simulink model "project_sim"  (R2022b)
settings: Solver=VariableStepAuto  StartTime=0.0  StopTime=Tf  RelTol=1e-3
values from neighbouring files (symbols this model uses):
  FSW_freq = 1/10    (= 0.1)    [project.m]
  h0 = 4881    [project.m]
  J = J + J'    [TestRK4.m]    (also in project.m = 1E-4*[24181836 3783405 3898808)
  kd_nonlin = 10    [project.m]
  kp_nonlin = 0.1    [project.m]
  mu = 398600    [project.m]
  Phat0 = blkdiag(1E-3*eye(3),1E-4*eye(3))    [project.m]
  Q_filter = blkdiag(1E-8*eye(3),0.1*w_noise_scale*eye(3))    [project.m]
  q_inertial2body_0_est = QuatProduct(dq0_disp,q_inertial2body_0)    [project.m]
  q_inertial2body_0_true = QuatProduct(dq0,q_inertial2body_0_est)    [project.m]
  q_inertial2LVLH_0 = DCM2Quat(T_inertial2LVLH_0)    [project.m]
  q_LVLH2body_0_est = QuatProduct(q_inertial2body_0_est,QuatInv(q_inertial2LVLH_0))    [project.m]
  q_LVLH2body_f = QuatProduct(q_change,q_LVLH2body_0)    [project.m]
  rate_max = Inf*(pi/180)    (= inf)    [project.m]
  Sigma_a = 1E-3*eye(3)    [project.m]
  Sigma_w = 1E-3*eye(3)    [project.m]
  Tf_man = 200    [project.m]
  underweight = 0.5    [project.m]
  w_b_LVLH_man = dtheta_LVLH/Tf_man*dn_LVLH    [project.m]
  w_body_wrt_inertial_0_est = w_body_wrt_inertial_0 + init_disp(4:6)    [project.m]
  w_body_wrt_inertial_0_true = w_body_wrt_inertial_0_est + init_err(4:6)    [project.m]
  w_LVLH_wrt_inertial_in_LVLH = [0, -n, 0]'    [project.m]
undefined symbols (not defined in the file or in its folder): r_inertial_0, v_inertial_0
settings Model: SimulationMode=rapid-accelerator  Creator=corey  LastModifiedBy=cm58349
settings DebuggingCC: UnconnectedInputMsg=warning  UnconnectedOutputMsg=warning  UnconnectedLineMsg=warning
settings ModelReferenceCC: EnableRefExpFcnMdlSchedulingChecks=on
settings RTWCC: DLArmComputeVersion=19.05

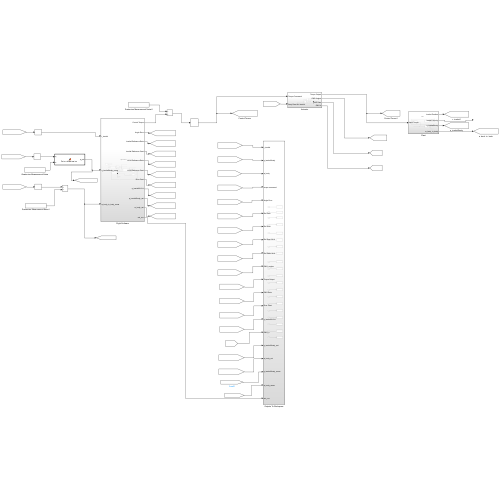
[thumbnail: Simulink's stored preview of the top-level diagram]
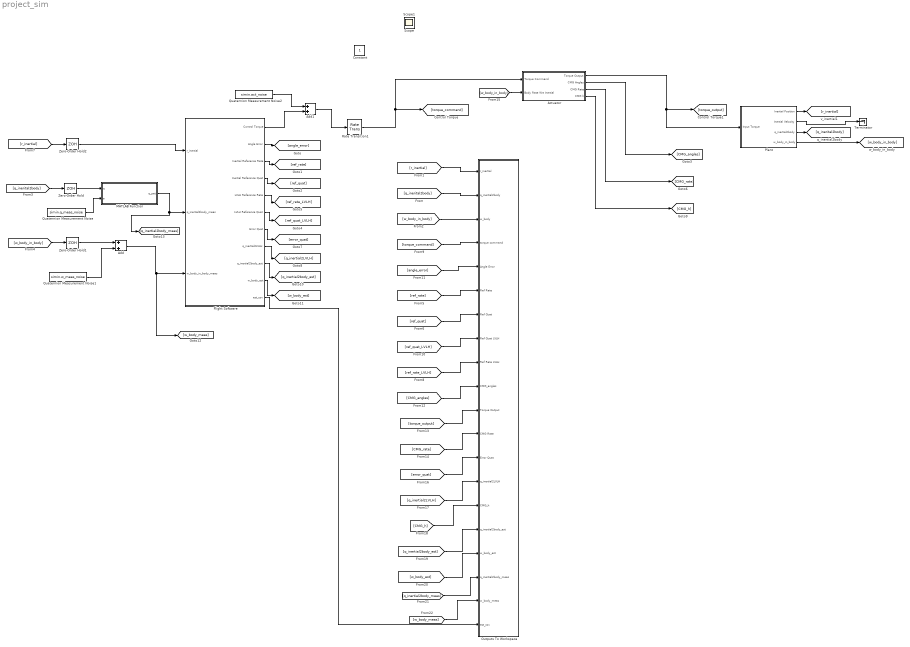
== system project_sim ==
  Actuator : Subsystem
  Add : Sum
  Add1 : Sum
  Flight Software : Subsystem
  MATLAB Function : MATLAB Function  TreatAsAtomicUnit=on
  Outputs To Workspace : Subsystem
  Plant : Subsystem
  Quaternion Measurement Noise : FromWorkspace  VariableName=simin.q_meas_noise  SampleTime=FSW_freq
  Quaternion Measurement Noise1 : FromWorkspace  VariableName=simin.w_meas_noise  SampleTime=FSW_freq
  Quaternion Measurement Noise2 : FromWorkspace  VariableName=simin.act_noise  SampleTime=FSW_freq
  Rate Transition1 : RateTransition
  Terminator : Terminator
  Zero-Order Hold : ZeroOrderHold  SampleTime=FSW_freq
  Zero-Order Hold1 : ZeroOrderHold  SampleTime=FSW_freq
  Zero-Order Hold2 : ZeroOrderHold  SampleTime=FSW_freq
  Constant : Constant  IOType=siggen
  Scope : Scope
  Scope1 : Scope
  wires:
  Plant/4(w_body_in_body) -> [w_body_in_body]
  Plant/3(q_inertial2body) -> [q_inerital2body]
  Plant/2(Inertial Velocity) -> Terminator/1
  Plant/1(Inertial Position) -> [r_inertial]
  [q_inerital2body] -> Outputs To Workspace/2(q_inertial2body)
  [w_body_in_body] -> Outputs To Workspace/3(w_body)
  [r_inertial] -> Outputs To Workspace/1(r_inertial)
  [torque_command] -> Outputs To Workspace/4(torque command)
  [angle_error] -> Outputs To Workspace/5(Angle Error)
  Flight Software/2(Angle Error) -> [angle_error]
  Flight Software/3(Inertial Reference Rate) -> [ref_rate]
  Flight Software/4(Inertial Reference Quat) -> [ref_quat]
  [ref_rate] -> Outputs To Workspace/6(Ref Rate)
  [ref_quat] -> Outputs To Workspace/7(Ref Quat)
  [ref_rate_LVLH] -> Outputs To Workspace/9(Ref Rate LVLH)
  [ref_quat_LVLH] -> Outputs To Workspace/8(Ref Quat LVLH)
  Flight Software/5(LVLH Reference Rate) -> [ref_rate_LVLH]
  Flight Software/6(LVLH Reference Quat) -> [ref_quat_LVLH]
  [CMG_angles] -> Outputs To Workspace/10(CMG_angles)
  [torque_output] -> Outputs To Workspace/11(Torque Output)
  [CMG_rate] -> Outputs To Workspace/12(CMG Rate)
  Actuator/1(Torque Output) -> Plant/1(Input Torque), [torque_output]
  Actuator/2(CMG Angles) -> [CMG_angles]
  Actuator/3(CMG Rate) -> [CMG_rate]
  [w_body_in_body] -> Actuator/2(Body Rate Wrt Inertial)
  Flight Software/7(Error Quat) -> [error_quat]
  [error_quat] -> Outputs To Workspace/13(Error Quat)
  Flight Software/8(q_inertial2LVLH) -> [q_inertial2LVLH]
  [q_inertial2LVLH] -> Outputs To Workspace/14(q_inertial2LVLH)
  Actuator/4(CMG h) -> [CMG_h]
  [CMG_h] -> Outputs To Workspace/15(CMG_h)
  [q_inerital2body] -> Zero-Order Hold/1
  [w_body_in_body] -> Zero-Order Hold1/1
  [r_inertial] -> Zero-Order Hold2/1
  Zero-Order Hold2/1 -> Flight Software/1(r_inertial)
  Rate Transition1/1 -> Actuator/1(Torque Command), [torque_command]
  Zero-Order Hold/1 -> MATLAB Function/1(q)
  MATLAB Function/1(q_pet) -> [q_inertial2body_meas], Flight Software/2(q_inertial2body_meas)
  Quaternion Measurement Noise/1 -> MATLAB Function/2(a)
  Flight Software/9(q_inertial2body_est) -> [q_inertial2body_est]
  Flight Software/10(w_body_est) -> [w_body_est]
  [q_inertial2body_est] -> Outputs To Workspace/16(q_inertial2body_est)
  [w_body_est] -> Outputs To Workspace/17(w_body_est)
  Zero-Order Hold1/1 -> Add/1
  Add/1 -> [w_body_meas], Flight Software/3(w_body_in_body_meas)
  Quaternion Measurement Noise1/1 -> Add/2
  [q_inertial2body_meas] -> Outputs To Workspace/18(q_inertial2body_meas)
  [w_body_meas] -> Outputs To Workspace/19(w_body_meas)
  Add1/1 -> Rate Transition1/1
  Flight Software/1(Control Torque) -> Add1/2
  Quaternion Measurement Noise2/1 -> Add1/1
  Flight Software/11(est_cov) -> Outputs To Workspace/20(est_cov)

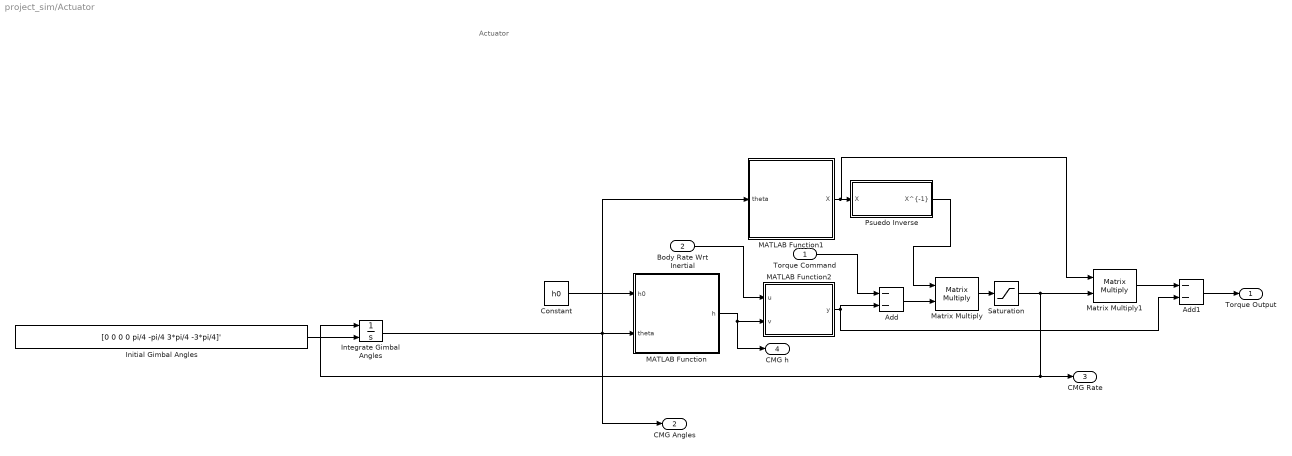
== system project_sim/Actuator ==
  note: Actuator
  Torque Command : Inport
  Body Rate Wrt Inertial : Inport  Port=2
  Add : Sum  Inputs=--
  Add1 : Sum  Inputs=--
  Constant : Constant  Value=h0
  Initial Gimbal Angles : Constant  Value=[0 0 0 0 pi/4 -pi/4 3*pi/4 -3*pi/4]'
  Integrate Gimbal Angles : Integrator  InitialConditionSource=external
  MATLAB Function : MATLAB Function  TreatAsAtomicUnit=on
  MATLAB Function1 : MATLAB Function  TreatAsAtomicUnit=on
  MATLAB Function2 : MATLAB Function  TreatAsAtomicUnit=on
  Matrix Multiply : Product  Multiplication=Matrix(*)
  Matrix Multiply1 : Product  Multiplication=Matrix(*)
  Psuedo Inverse : Subsystem
  Saturation : Saturate  UpperLimit=rate_max  LowerLimit=-1*rate_max
  Torque Output : Outport
  CMG Angles : Outport  Port=2
  CMG Rate : Outport  Port=3
  CMG h : Outport  Port=4
  wires:
  Initial Gimbal Angles/1 -> Integrate Gimbal Angles/2
  Constant/1 -> MATLAB Function/1(h0)
  MATLAB Function2/1(y) -> Add/2, Add1/2
  Torque Command/1 -> Add/1
  Body Rate Wrt Inertial/1 -> MATLAB Function2/1(u)
  MATLAB Function/1(h) -> MATLAB Function2/2(v), CMG h/1
  MATLAB Function1/1(X) -> Matrix Multiply1/1, Psuedo Inverse/1(X)
  Psuedo Inverse/1("X^{-1}") -> Matrix Multiply/1
  Add/1 -> Matrix Multiply/2
  Matrix Multiply1/1 -> Add1/1
  Add1/1 -> Torque Output/1
  Integrate Gimbal Angles/1 -> MATLAB Function/2(theta), CMG Angles/1, MATLAB Function1/1(theta)
  Matrix Multiply/1 -> Saturation/1
  Saturation/1 -> Integrate Gimbal Angles/1, CMG Rate/1, Matrix Multiply1/2

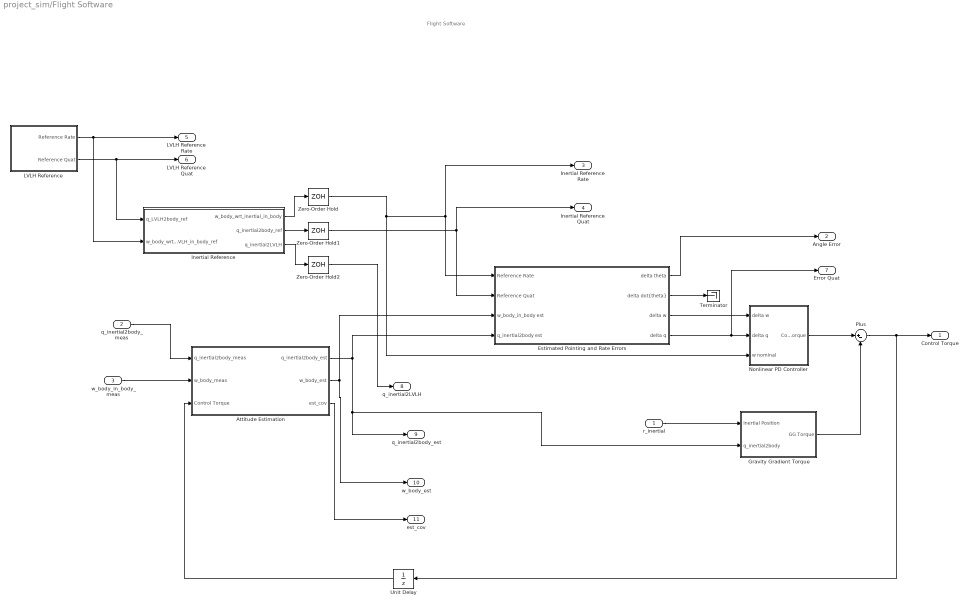
== system project_sim/Flight Software ==
  note: Flight Software
  r_inertial : Inport
  q_inertial2body_meas : Inport  Port=2
  w_body_in_body_meas : Inport  Port=3
  Attitude Estimation : Subsystem
  Estimated Pointing and Rate Errors : Subsystem
  Gravity Gradient Torque : Subsystem
  Inertial Reference : Subsystem
  LVLH Reference : Subsystem
  Nonlinear PD Controller : Subsystem
  Plus : Sum  Inputs=|+-
  Terminator : Terminator
  Unit Delay : UnitDelay  InitialCondition=[0 0 0]'  SampleTime=-1  HasFrameUpgradeWarning=on
  Zero-Order Hold : ZeroOrderHold  SampleTime=FSW_freq
  Zero-Order Hold1 : ZeroOrderHold  SampleTime=FSW_freq
  Zero-Order Hold2 : ZeroOrderHold  SampleTime=FSW_freq
  Control Torque : Outport
  Angle Error : Outport  Port=2
  Inertial Reference Rate : Outport  Port=3
  Inertial Reference Quat : Outport  Port=4
  LVLH Reference Rate : Outport  Port=5
  LVLH Reference Quat : Outport  Port=6
  Error Quat : Outport  Port=7
  q_inertial2LVLH : Outport  Port=8
  q_inertial2body_est : Outport  Port=9
  w_body_est : Outport  Port=10
  est_cov : Outport  Port=11
  wires:
  Estimated Pointing and Rate Errors/1(delta theta) -> Angle Error/1
  Inertial Reference/1(w_body_wrt_inertial_in_body) -> Zero-Order Hold/1
  Inertial Reference/2(q_inertial2body_ref) -> Zero-Order Hold1/1
  LVLH Reference/1(Reference Rate) -> Inertial Reference/2(w_body_wrt_LVLH_in_body_ref), LVLH Reference Rate/1
  LVLH Reference/2(Reference Quat) -> Inertial Reference/1(q_LVLH2body_ref), LVLH Reference Quat/1
  Estimated Pointing and Rate Errors/3(delta w) -> Nonlinear PD Controller/1(delta w)
  Estimated Pointing and Rate Errors/4(delta q) -> Error Quat/1, Nonlinear PD Controller/2(delta q)
  Estimated Pointing and Rate Errors/2("delta dot{theta}") -> Terminator/1
  Nonlinear PD Controller/1(Control Torque) -> Plus/1
  Plus/1 -> Unit Delay/1, Control Torque/1
  Gravity Gradient Torque/1(GG Torque) -> Plus/2
  r_inertial/1 -> Gravity Gradient Torque/1(Inertial Position)
  Inertial Reference/3(q_inertial2LVLH) -> Zero-Order Hold2/1
  Zero-Order Hold/1 -> Nonlinear PD Controller/3(w nominal), Inertial Reference Rate/1, Estimated Pointing and Rate Errors/1(Reference Rate)
  Zero-Order Hold1/1 -> Inertial Reference Quat/1, Estimated Pointing and Rate Errors/2(Reference Quat)
  Zero-Order Hold2/1 -> q_inertial2LVLH/1
  q_inertial2body_meas/1 -> Attitude Estimation/1(q_inertial2body_meas)
  Attitude Estimation/1(q_inertial2body_est) -> Gravity Gradient Torque/2(q_inertial2body), q_inertial2body_est/1, Estimated Pointing and Rate Errors/4(q_inertial2body est)
  Attitude Estimation/2(w_body_est) -> w_body_est/1, Estimated Pointing and Rate Errors/3(w_body_in_body est)
  w_body_in_body_meas/1 -> Attitude Estimation/2(w_body_meas)
  Unit Delay/1 -> Attitude Estimation/3(Control Torque)
  Attitude Estimation/3(est_cov) -> est_cov/1

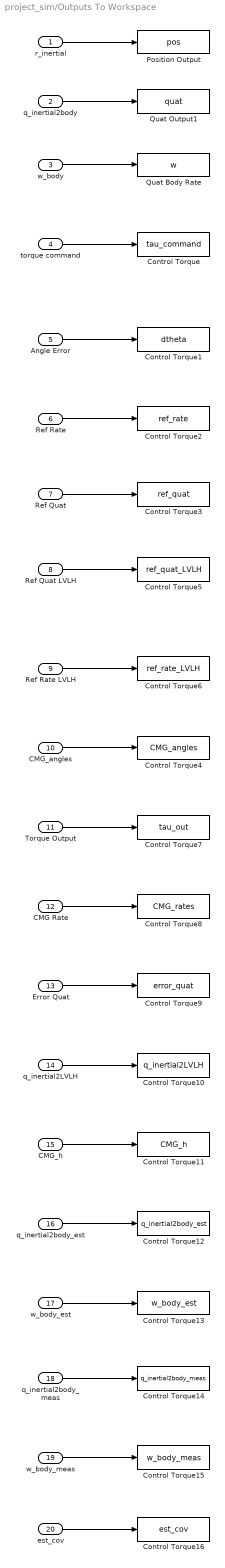
== system project_sim/Outputs To Workspace ==
  r_inertial : Inport
  q_inertial2body : Inport  Port=2
  w_body : Inport  Port=3
  torque command : Inport  Port=4
  Angle Error : Inport  Port=5
  Ref Rate : Inport  Port=6
  Ref Quat : Inport  Port=7
  Ref Quat LVLH : Inport  Port=8
  Ref Rate LVLH : Inport  Port=9
  CMG_angles : Inport  Port=10
  Torque Output : Inport  Port=11
  CMG Rate : Inport  Port=12
  Error Quat : Inport  Port=13
  q_inertial2LVLH : Inport  Port=14
  CMG_h : Inport  Port=15
  q_inertial2body_est : Inport  Port=16
  w_body_est : Inport  Port=17
  q_inertial2body_meas : Inport  Port=18
  w_body_meas : Inport  Port=19
  est_cov : Inport  Port=20
  Control Torque : ToWorkspace  VariableName=tau_command  SaveFormat=Timeseries  SampleTime=FSW_freq
  Control Torque1 : ToWorkspace  VariableName=dtheta  SaveFormat=Timeseries  SampleTime=FSW_freq
  Control Torque10 : ToWorkspace  VariableName=q_inertial2LVLH  SaveFormat=Timeseries  SampleTime=FSW_freq
  Control Torque11 : ToWorkspace  VariableName=CMG_h  SaveFormat=Timeseries  SampleTime=FSW_freq
  Control Torque12 : ToWorkspace  VariableName=q_inertial2body_est  SaveFormat=Timeseries  SampleTime=FSW_freq
  Control Torque13 : ToWorkspace  VariableName=w_body_est  SaveFormat=Timeseries  SampleTime=FSW_freq
  Control Torque14 : ToWorkspace  VariableName=q_inertial2body_meas  SaveFormat=Timeseries  SampleTime=FSW_freq
  Control Torque15 : ToWorkspace  VariableName=w_body_meas  SaveFormat=Timeseries  SampleTime=FSW_freq
  Control Torque16 : ToWorkspace  VariableName=est_cov  SaveFormat=Timeseries  SampleTime=FSW_freq
  Control Torque2 : ToWorkspace  VariableName=ref_rate  SaveFormat=Timeseries  SampleTime=FSW_freq
  Control Torque3 : ToWorkspace  VariableName=ref_quat  SaveFormat=Timeseries  SampleTime=FSW_freq
  Control Torque4 : ToWorkspace  VariableName=CMG_angles  SaveFormat=Timeseries  SampleTime=FSW_freq
  Control Torque5 : ToWorkspace  VariableName=ref_quat_LVLH  SaveFormat=Timeseries  SampleTime=FSW_freq
  Control Torque6 : ToWorkspace  VariableName=ref_rate_LVLH  SaveFormat=Timeseries  SampleTime=FSW_freq
  Control Torque7 : ToWorkspace  VariableName=tau_out  SaveFormat=Timeseries  SampleTime=FSW_freq
  Control Torque8 : ToWorkspace  VariableName=CMG_rates  SaveFormat=Timeseries  SampleTime=FSW_freq
  Control Torque9 : ToWorkspace  VariableName=error_quat  SaveFormat=Timeseries  SampleTime=FSW_freq
  Position Output : ToWorkspace  VariableName=pos  SaveFormat=Timeseries  SampleTime=FSW_freq
  Quat Body Rate : ToWorkspace  VariableName=w  SaveFormat=Timeseries  SampleTime=FSW_freq
  Quat Output1 : ToWorkspace  VariableName=quat  SaveFormat=Timeseries  SampleTime=FSW_freq
  wires:
  r_inertial/1 -> Position Output/1
  w_body/1 -> Quat Body Rate/1
  q_inertial2body/1 -> Quat Output1/1
  torque command/1 -> Control Torque/1
  Angle Error/1 -> Control Torque1/1
  Ref Rate/1 -> Control Torque2/1
  Ref Quat/1 -> Control Torque3/1
  Ref Quat LVLH/1 -> Control Torque5/1
  Ref Rate LVLH/1 -> Control Torque6/1
  CMG_angles/1 -> Control Torque4/1
  Torque Output/1 -> Control Torque7/1
  CMG Rate/1 -> Control Torque8/1
  Error Quat/1 -> Control Torque9/1
  q_inertial2LVLH/1 -> Control Torque10/1
  CMG_h/1 -> Control Torque11/1
  w_body_est/1 -> Control Torque13/1
  q_inertial2body_est/1 -> Control Torque12/1
  q_inertial2body_meas/1 -> Control Torque14/1
  w_body_meas/1 -> Control Torque15/1
  est_cov/1 -> Control Torque16/1

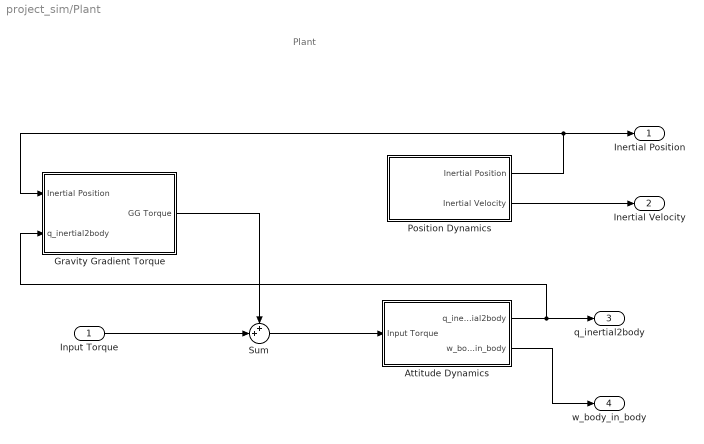
== system project_sim/Plant ==
  note: Plant
  Input Torque : Inport
  Attitude Dynamics : Subsystem
  Gravity Gradient Torque : Subsystem
  Position Dynamics : Subsystem
  Sum : Sum  Inputs=++|
  Inertial Position : Outport
  Inertial Velocity : Outport  Port=2
  q_inertial2body : Outport  Port=3
  w_body_in_body : Outport  Port=4
  wires:
  Position Dynamics/1(Inertial Position) -> Gravity Gradient Torque/1(Inertial Position), Inertial Position/1
  Position Dynamics/2(Inertial Velocity) -> Inertial Velocity/1
  Attitude Dynamics/1(q_inertial2body) -> Gravity Gradient Torque/2(q_inertial2body), q_inertial2body/1
  Attitude Dynamics/2(w_body_in_body) -> w_body_in_body/1
  Input Torque/1 -> Sum/2
  Sum/1 -> Attitude Dynamics/1(Input Torque)
  Gravity Gradient Torque/1(GG Torque) -> Sum/1

== system project_sim/Actuator/Psuedo Inverse ==
  X : Inport
  Matrix Divide : Product  Inputs=*/  Multiplication=Matrix(*)
  Matrix Multiply : Product  Multiplication=Matrix(*)
  Transpose : Math  Operator=transpose
  "X^{-1}" : Outport
  wires:
  Transpose/1 -> Matrix Divide/1, Matrix Multiply/2
  X/1 -> Transpose/1, Matrix Multiply/1
  Matrix Multiply/1 -> Matrix Divide/2
  Matrix Divide/1 -> "X^{-1}"/1

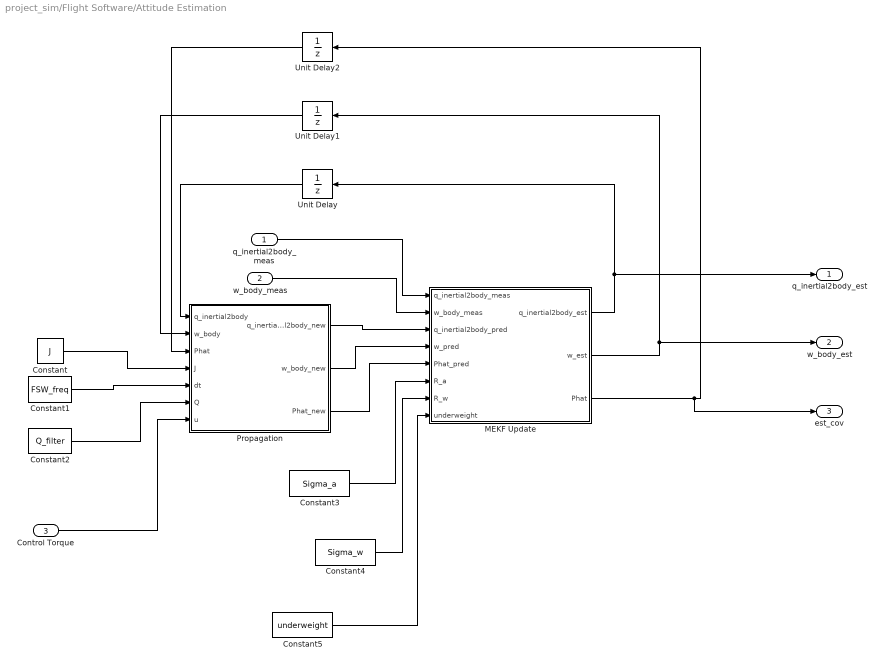
== system project_sim/Flight Software/Attitude Estimation ==
  q_inertial2body_meas : Inport
  w_body_meas : Inport  Port=2
  Control Torque : Inport  Port=3
  Constant : Constant  Value=J
  Constant1 : Constant  Value=FSW_freq
  Constant2 : Constant  Value=Q_filter
  Constant3 : Constant  Value=Sigma_a
  Constant4 : Constant  Value=Sigma_w
  Constant5 : Constant  Value=underweight
  MEKF Update : MATLAB Function  TreatAsAtomicUnit=on
  Propagation : MATLAB Function  TreatAsAtomicUnit=on
  Unit Delay : UnitDelay  InitialCondition=q_inertial2body_0_est  SampleTime=-1  HasFrameUpgradeWarning=on
  Unit Delay1 : UnitDelay  InitialCondition=w_body_wrt_inertial_0_est  SampleTime=-1  HasFrameUpgradeWarning=on
  Unit Delay2 : UnitDelay  InitialCondition=Phat0  SampleTime=-1  HasFrameUpgradeWarning=on
  q_inertial2body_est : Outport
  w_body_est : Outport  Port=2
  est_cov : Outport  Port=3
  wires:
  q_inertial2body_meas/1 -> MEKF Update/1(q_inertial2body_meas)
  Constant/1 -> Propagation/4(J)
  Constant1/1 -> Propagation/5(dt)
  Constant2/1 -> Propagation/6(Q)
  Unit Delay2/1 -> Propagation/3(Phat)
  MEKF Update/2(w_est) -> w_body_est/1, Unit Delay1/1
  Unit Delay1/1 -> Propagation/2(w_body)
  MEKF Update/1(q_inertial2body_est) -> q_inertial2body_est/1, Unit Delay/1
  Unit Delay/1 -> Propagation/1(q_inertial2body)
  Propagation/1(q_inertial2body_new) -> MEKF Update/3(q_inertial2body_pred)
  Propagation/2(w_body_new) -> MEKF Update/4(w_pred)
  Propagation/3(Phat_new) -> MEKF Update/5(Phat_pred)
  Constant3/1 -> MEKF Update/6(R_a)
  Constant4/1 -> MEKF Update/7(R_w)
  w_body_meas/1 -> MEKF Update/2(w_body_meas)
  MEKF Update/3(Phat) -> est_cov/1, Unit Delay2/1
  Control Torque/1 -> Propagation/7(u)
  Constant5/1 -> MEKF Update/8(underweight)

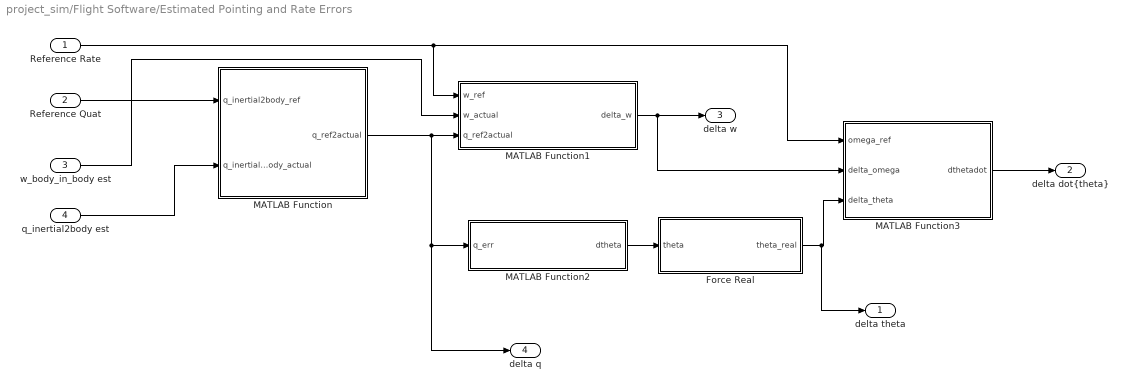
== system project_sim/Flight Software/Estimated Pointing and Rate Errors ==
  Reference Rate : Inport
  Reference Quat : Inport  Port=2
  w_body_in_body est : Inport  Port=3
  q_inertial2body est : Inport  Port=4
  Force Real : MATLAB Function  TreatAsAtomicUnit=on
  MATLAB Function : MATLAB Function  TreatAsAtomicUnit=on
  MATLAB Function1 : MATLAB Function  TreatAsAtomicUnit=on
  MATLAB Function2 : MATLAB Function  TreatAsAtomicUnit=on
  MATLAB Function3 : MATLAB Function  TreatAsAtomicUnit=on
  delta theta : Outport
  "delta dot{theta}" : Outport  Port=2
  delta w : Outport  Port=3
  delta q : Outport  Port=4
  wires:
  Reference Quat/1 -> MATLAB Function/1(q_inertial2body_ref)
  q_inertial2body est/1 -> MATLAB Function/2(q_inertial2body_actual)
  MATLAB Function/1(q_ref2actual) -> delta q/1, MATLAB Function2/1(q_err), MATLAB Function1/3(q_ref2actual)
  Reference Rate/1 -> MATLAB Function3/1(omega_ref), MATLAB Function1/1(w_ref)
  w_body_in_body est/1 -> MATLAB Function1/2(w_actual)
  MATLAB Function3/1(dthetadot) -> "delta dot{theta}"/1
  MATLAB Function2/1(dtheta) -> Force Real/1(theta)
  Force Real/1(theta_real) -> delta theta/1, MATLAB Function3/3(delta_theta)
  MATLAB Function1/1(delta_w) -> delta w/1, MATLAB Function3/2(delta_omega)

== system project_sim/Flight Software/Gravity Gradient Torque ==
  Inertial Position : Inport
  q_inertial2body : Inport  Port=2
  GG Torque Computation : MATLAB Function  TreatAsAtomicUnit=on
  Gravity Constant : Constant  Value=mu
  Inerita Matrix : Constant  Value=J
  MATLAB Function : MATLAB Function  TreatAsAtomicUnit=on
  GG Torque : Outport
  wires:
  Inerita Matrix/1 -> GG Torque Computation/1(J)
  Inertial Position/1 -> MATLAB Function/2(r), GG Torque Computation/3(r_inertial)
  q_inertial2body/1 -> GG Torque Computation/4(q_inertial2body)
  GG Torque Computation/1(T) -> GG Torque/1
  Gravity Constant/1 -> MATLAB Function/1(mu)
  MATLAB Function/1(n) -> GG Torque Computation/2(n)

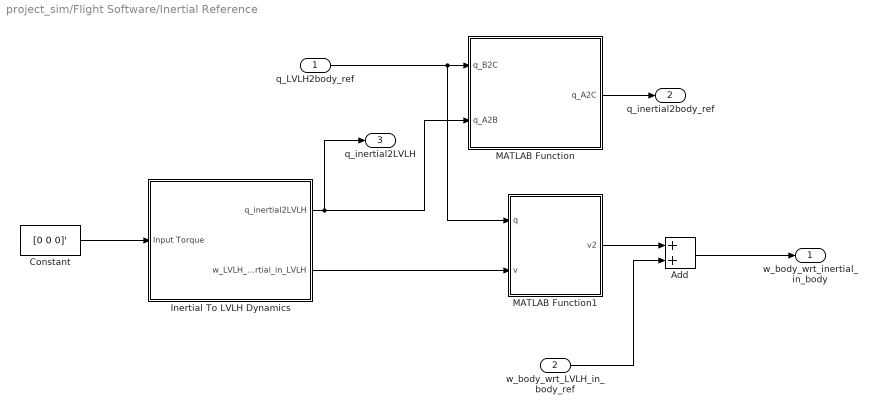
== system project_sim/Flight Software/Inertial Reference ==
  q_LVLH2body_ref : Inport
  w_body_wrt_LVLH_in_body_ref : Inport  Port=2
  Add : Sum
  Constant : Constant  Value=[0 0 0]'
  Inertial To LVLH Dynamics : Subsystem
  MATLAB Function : MATLAB Function  TreatAsAtomicUnit=on
  MATLAB Function1 : MATLAB Function  TreatAsAtomicUnit=on
  w_body_wrt_inertial_in_body : Outport
  q_inertial2body_ref : Outport  Port=2
  q_inertial2LVLH : Outport  Port=3
  wires:
  Constant/1 -> Inertial To LVLH Dynamics/1(Input Torque)
  Inertial To LVLH Dynamics/1(q_inertial2LVLH) -> MATLAB Function/2(q_A2B), q_inertial2LVLH/1
  MATLAB Function/1(q_A2C) -> q_inertial2body_ref/1
  q_LVLH2body_ref/1 -> MATLAB Function1/1(q), MATLAB Function/1(q_B2C)
  Inertial To LVLH Dynamics/2(w_LVLH_wrt_inertial_in_LVLH) -> MATLAB Function1/2(v)
  MATLAB Function1/1(v2) -> Add/1
  Add/1 -> w_body_wrt_inertial_in_body/1
  w_body_wrt_LVLH_in_body_ref/1 -> Add/2

== system project_sim/Flight Software/LVLH Reference ==
  Attitude Hold : Subsystem  TreatAsAtomicUnit=on
  Attitude Slew : Subsystem  TreatAsAtomicUnit=on
  Clock : Clock
  If : If  IfExpression=u1 < Tf_man
  Merge : Merge
  Merge1 : Merge
  Reference Rate : Outport
  Reference Quat : Outport  Port=2
  wires:
  Clock/1 -> If/1
  If/1 -> Attitude Slew/Action
  If/2 -> Attitude Hold/Action
  Attitude Slew/1(q_LVLH2body) -> Merge/1
  Attitude Hold/1(q_inertial2body) -> Merge/2
  Merge/1 -> Reference Quat/1
  Merge1/1 -> Reference Rate/1
  Attitude Slew/2(w_body_in_body) -> Merge1/1
  Attitude Hold/2(w_body) -> Merge1/2

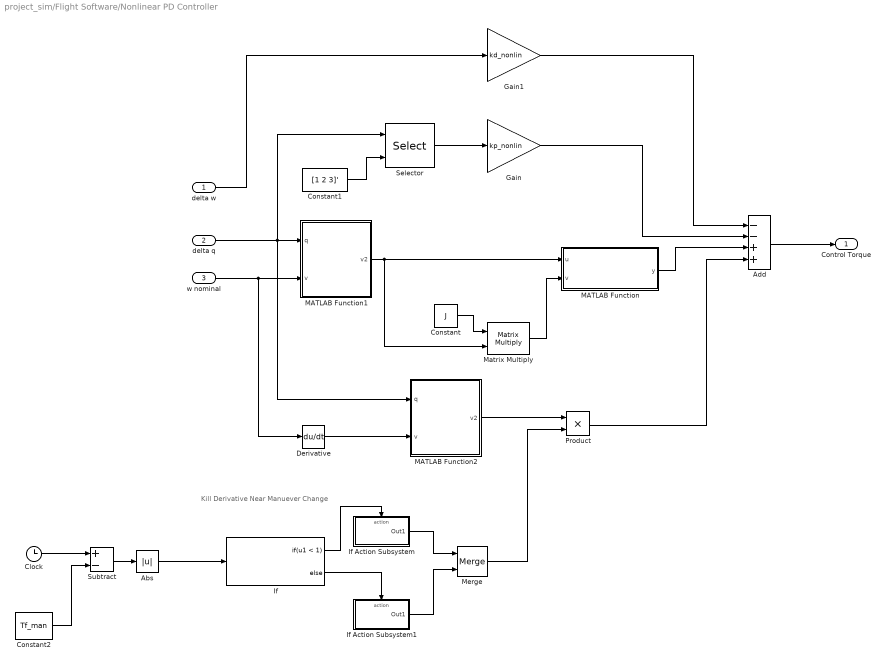
== system project_sim/Flight Software/Nonlinear PD Controller ==
  note: Kill Derivative Near Manuever Change
  delta w : Inport
  delta q : Inport  Port=2
  w nominal : Inport  Port=3
  Abs : Abs  SaturateOnIntegerOverflow=off
  Add : Sum  Inputs=--++
  Clock : Clock
  Constant : Constant  Value=J
  Constant1 : Constant  Value=[1 2 3]'
  Constant2 : Constant  Value=Tf_man
  Derivative : Derivative  CoefficientInTFapproximation=Inf
  Gain : Gain  Gain=kp_nonlin
  Gain1 : Gain  Gain=kd_nonlin
  If : If  IfExpression=u1 < 1
  If Action Subsystem : Subsystem  TreatAsAtomicUnit=on
  If Action Subsystem1 : Subsystem  TreatAsAtomicUnit=on
  MATLAB Function : MATLAB Function  TreatAsAtomicUnit=on
  MATLAB Function1 : MATLAB Function  TreatAsAtomicUnit=on
  MATLAB Function2 : MATLAB Function  TreatAsAtomicUnit=on
  Matrix Multiply : Product  Multiplication=Matrix(*)
  Merge : Merge
  Product : Product
  Selector : Selector  InputPortWidth=4  IndexOptions=Index vector (port)  Indices=[1 3]  OutputSizes=1
  Subtract : Sum  Inputs=+-
  Control Torque : Outport
  wires:
  delta q/1 -> Selector/1, MATLAB Function2/1(q), MATLAB Function1/1(q)
  w nominal/1 -> Derivative/1, MATLAB Function1/2(v)
  MATLAB Function1/1(v2) -> MATLAB Function/1(u), Matrix Multiply/2
  Constant/1 -> Matrix Multiply/1
  Matrix Multiply/1 -> MATLAB Function/2(v)
  Derivative/1 -> MATLAB Function2/2(v)
  Add/1 -> Control Torque/1
  Constant1/1 -> Selector/2
  Selector/1 -> Gain/1
  Gain/1 -> Add/2
  delta w/1 -> Gain1/1
  Gain1/1 -> Add/1
  MATLAB Function2/1(v2) -> Product/1
  Product/1 -> Add/4
  MATLAB Function/1(y) -> Add/3
  If/1 -> If Action Subsystem/Action
  If/2 -> If Action Subsystem1/Action
  Clock/1 -> Subtract/1
  Constant2/1 -> Subtract/2
  Subtract/1 -> Abs/1
  Abs/1 -> If/1
  If Action Subsystem/1(Out1) -> Merge/1
  If Action Subsystem1/1(Out1) -> Merge/2
  Merge/1 -> Product/2

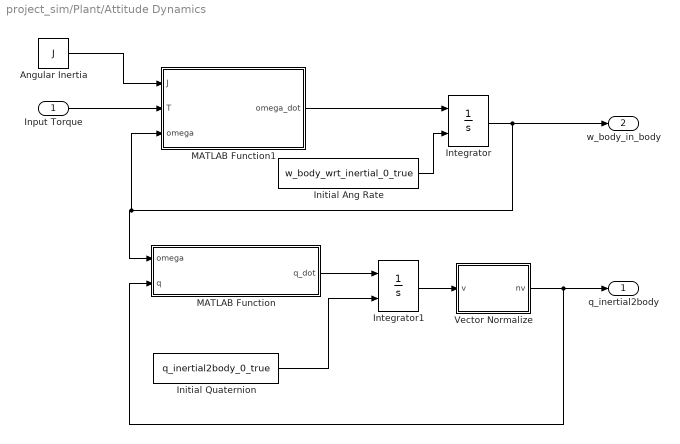
== system project_sim/Plant/Attitude Dynamics ==
  Input Torque : Inport
  Angular Inertia : Constant  Value=J
  Initial Ang Rate : Constant  Value=w_body_wrt_inertial_0_true
  Initial Quaternion : Constant  Value=q_inertial2body_0_true
  Integrator : Integrator  InitialConditionSource=external
  Integrator1 : Integrator  InitialConditionSource=external
  MATLAB Function : MATLAB Function  TreatAsAtomicUnit=on
  MATLAB Function1 : MATLAB Function  TreatAsAtomicUnit=on
  Vector Normalize : MATLAB Function  TreatAsAtomicUnit=on
  q_inertial2body : Outport
  w_body_in_body : Outport  Port=2
  wires:
  Integrator/1 -> MATLAB Function1/3(omega), MATLAB Function/1(omega), w_body_in_body/1
  MATLAB Function1/1(omega_dot) -> Integrator/1
  Initial Ang Rate/1 -> Integrator/2
  MATLAB Function/1(q_dot) -> Integrator1/1
  Initial Quaternion/1 -> Integrator1/2
  Integrator1/1 -> Vector Normalize/1(v)
  Vector Normalize/1(nv) -> MATLAB Function/2(q), q_inertial2body/1
  Input Torque/1 -> MATLAB Function1/2(T)
  Angular Inertia/1 -> MATLAB Function1/1(J)

== system project_sim/Plant/Gravity Gradient Torque ==
  Inertial Position : Inport
  q_inertial2body : Inport  Port=2
  GG Torque Computation : MATLAB Function  TreatAsAtomicUnit=on
  Gravity Constant : Constant  Value=mu
  Inerita Matrix : Constant  Value=J
  MATLAB Function : MATLAB Function  TreatAsAtomicUnit=on
  GG Torque : Outport
  wires:
  Inerita Matrix/1 -> GG Torque Computation/1(J)
  Inertial Position/1 -> MATLAB Function/2(r), GG Torque Computation/3(r_inertial)
  q_inertial2body/1 -> GG Torque Computation/4(q_inertial2body)
  GG Torque Computation/1(T) -> GG Torque/1
  Gravity Constant/1 -> MATLAB Function/1(mu)
  MATLAB Function/1(n) -> GG Torque Computation/2(n)

== system project_sim/Plant/Position Dynamics ==
  Gravity Constant : Constant  Value=mu
  Initial Position : Constant  Value=r_inertial_0
  Initial Velocity : Constant  Value=v_inertial_0
  Integrator : Integrator  InitialConditionSource=external  InitialCondition=[6871, 0, 0]'
  Integrator1 : Integrator  InitialConditionSource=external  InitialCondition=[0, 7.6166, 0]'
  Vector Norm : MATLAB Function  TreatAsAtomicUnit=on
  Inertial Position : Outport
  Inertial Velocity : Outport  Port=2
  wires:
  Integrator/1 -> Vector Norm/1(r), Inertial Position/1  "Position"
  Integrator1/1 -> Inertial Velocity/1, Integrator/1  "Velocity"
  Vector Norm/1(a) -> Integrator1/1  "Accel"
  Gravity Constant/1 -> Vector Norm/2(mu)
  Initial Velocity/1 -> Integrator1/2
  Initial Position/1 -> Integrator/2

== system project_sim/Flight Software/Inertial Reference/Inertial To LVLH Dynamics ==
  Input Torque : Inport
  Attitude Dynamics : Subsystem
  q_inertial2LVLH : Outport
  w_LVLH_wrt_inertial_in_LVLH : Outport  Port=2
  wires:
  Input Torque/1 -> Attitude Dynamics/1(Input Torque)
  Attitude Dynamics/1(q_LVLH2body) -> q_inertial2LVLH/1
  Attitude Dynamics/2(w_body_in_body) -> w_LVLH_wrt_inertial_in_LVLH/1

== system project_sim/Flight Software/LVLH Reference/Attitude Hold ==
  Action Port : ActionPort  ActionPortLabel=else
  Constant : Constant  Value=q_LVLH2body_f
  Constant1 : Constant  Value=[0 0 0]'
  q_inertial2body : Outport
  w_body : Outport  Port=2
  wires:
  Constant/1 -> q_inertial2body/1
  Constant1/1 -> w_body/1

== system project_sim/Flight Software/LVLH Reference/Attitude Slew ==
  Action Port : ActionPort  ActionPortLabel=if(u1 < Tf_man)
  Constant : Constant  Value=[0 0 0]'
  Reference Plant : Subsystem
  q_LVLH2body : Outport
  w_body_in_body : Outport  Port=2
  wires:
  Constant/1 -> Reference Plant/1(Input Torque)
  Reference Plant/1(q_inertial2body) -> q_LVLH2body/1
  Reference Plant/2(w_body_in_body) -> w_body_in_body/1

== system project_sim/Flight Software/Nonlinear PD Controller/If Action Subsystem ==
  Action Port : ActionPort  ActionPortLabel=if(u1 < 1)
  Constant : Constant  Value=0
  Out1 : Outport
  wires:
  Constant/1 -> Out1/1

== system project_sim/Flight Software/Nonlinear PD Controller/If Action Subsystem1 ==
  Action Port : ActionPort  ActionPortLabel=else
  Constant : Constant
  Out1 : Outport
  wires:
  Constant/1 -> Out1/1

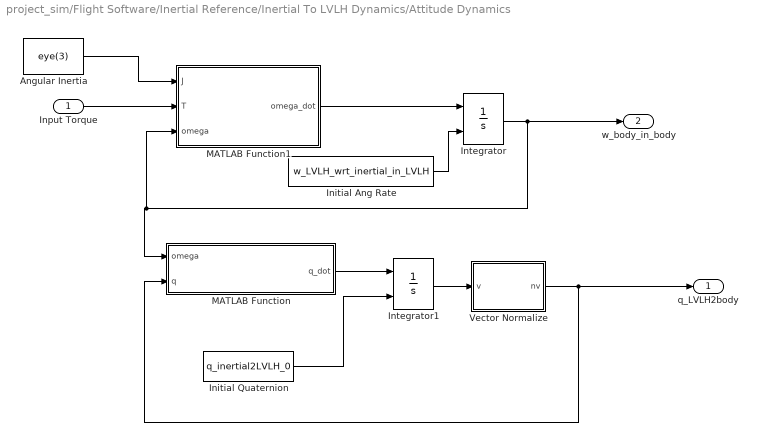
== system project_sim/Flight Software/Inertial Reference/Inertial To LVLH Dynamics/Attitude Dynamics ==
  Input Torque : Inport
  Angular Inertia : Constant  Value=eye(3)
  Initial Ang Rate : Constant  Value=w_LVLH_wrt_inertial_in_LVLH
  Initial Quaternion : Constant  Value=q_inertial2LVLH_0
  Integrator : Integrator  InitialConditionSource=external
  Integrator1 : Integrator  InitialConditionSource=external
  MATLAB Function : MATLAB Function  TreatAsAtomicUnit=on
  MATLAB Function1 : MATLAB Function  TreatAsAtomicUnit=on
  Vector Normalize : MATLAB Function  TreatAsAtomicUnit=on
  q_LVLH2body : Outport
  w_body_in_body : Outport  Port=2
  wires:
  Integrator/1 -> MATLAB Function1/3(omega), MATLAB Function/1(omega), w_body_in_body/1
  MATLAB Function1/1(omega_dot) -> Integrator/1
  Initial Ang Rate/1 -> Integrator/2
  MATLAB Function/1(q_dot) -> Integrator1/1
  Initial Quaternion/1 -> Integrator1/2
  Integrator1/1 -> Vector Normalize/1(v)
  Vector Normalize/1(nv) -> q_LVLH2body/1, MATLAB Function/2(q)
  Input Torque/1 -> MATLAB Function1/2(T)
  Angular Inertia/1 -> MATLAB Function1/1(J)

== system project_sim/Flight Software/LVLH Reference/Attitude Slew/Reference Plant ==
  Input Torque : Inport
  Attitude Dynamics : Subsystem
  q_inertial2body : Outport
  w_body_in_body : Outport  Port=2
  wires:
  Input Torque/1 -> Attitude Dynamics/1(Input Torque)
  Attitude Dynamics/1(q_LVLH2body) -> q_inertial2body/1
  Attitude Dynamics/2(w_body_in_body) -> w_body_in_body/1

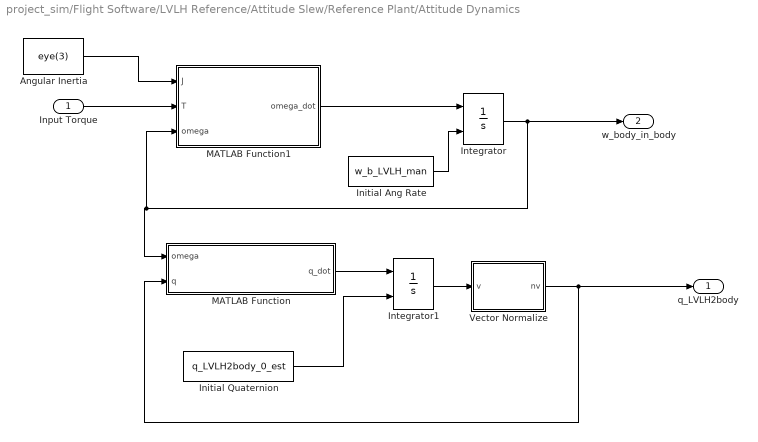
== system project_sim/Flight Software/LVLH Reference/Attitude Slew/Reference Plant/Attitude Dynamics ==
  Input Torque : Inport
  Angular Inertia : Constant  Value=eye(3)
  Initial Ang Rate : Constant  Value=w_b_LVLH_man
  Initial Quaternion : Constant  Value=q_LVLH2body_0_est
  Integrator : Integrator  InitialConditionSource=external
  Integrator1 : Integrator  InitialConditionSource=external
  MATLAB Function : MATLAB Function  TreatAsAtomicUnit=on
  MATLAB Function1 : MATLAB Function  TreatAsAtomicUnit=on
  Vector Normalize : MATLAB Function  TreatAsAtomicUnit=on
  q_LVLH2body : Outport
  w_body_in_body : Outport  Port=2
  wires:
  Integrator/1 -> MATLAB Function1/3(omega), MATLAB Function/1(omega), w_body_in_body/1
  MATLAB Function1/1(omega_dot) -> Integrator/1
  Initial Ang Rate/1 -> Integrator/2
  MATLAB Function/1(q_dot) -> Integrator1/1
  Initial Quaternion/1 -> Integrator1/2
  Integrator1/1 -> Vector Normalize/1(v)
  Vector Normalize/1(nv) -> q_LVLH2body/1, MATLAB Function/2(q)
  Input Torque/1 -> MATLAB Function1/2(T)
  Angular Inertia/1 -> MATLAB Function1/1(J)

== matlab function project_sim/Flight Software/Inertial Reference/MATLAB Function ==
  data: q_B2C input; q_A2C output; q_A2B input
function q_A2C = QuatProduct_sym(q_B2C,q_A2B)

q_A2C = QuatProduct(q_B2C,q_A2B);

== matlab function project_sim/Flight Software/LVLH Reference/Attitude Slew/Reference Plant/Attitude Dynamics/MATLAB Function ==
  data: omega input; q_dot output; q input
function q_dot = QuaternionEvolution(omega, q)
intermed = [omega; 0];
q_dot = 0.5*QuatProduct(intermed,q);

== matlab function project_sim/Flight Software/LVLH Reference/Attitude Slew/Reference Plant/Attitude Dynamics/MATLAB Function1 ==
  data: J input; omega_dot output; T input; omega input
function omega_dot = OmegaEvolution(J, T, omega)
omega_dot = J\(T - cross(omega, J*omega));

== matlab function project_sim/Flight Software/LVLH Reference/Attitude Slew/Reference Plant/Attitude Dynamics/Vector Normalize ==
  data: v input; nv output
function nv = NormVec(v)

nv = v/norm(v);

== matlab function project_sim/Flight Software/Nonlinear PD Controller/MATLAB Function1 ==
  data: q input; v2 output; v input
function v2 = QuatRotate_sym(q,v)

v2 = QuatTransform(q,v);

== matlab function project_sim/Flight Software/Estimated Pointing and Rate Errors/Force Real ==
  data: theta input; theta_real output
function theta_real = ForceReal(theta)

theta_real = real(theta);

== matlab function project_sim/Flight Software/Inertial Reference/MATLAB Function1 ==
  data: q input; v2 output; v input
function v2 = QuatRotate_sym(q,v)

v2 = QuatTransform(q,v);

== matlab function project_sim/Flight Software/Nonlinear PD Controller/MATLAB Function2 ==
  data: q input; v2 output; v input
function v2 = QuatRotate_sym(q,v)

v2 = QuatTransform(q,v);

== matlab function project_sim/Plant/Gravity Gradient Torque/GG Torque Computation ==
  data: J input; T output; n input; r_inertial input; q_inertial2body input
function T = GGTorque(J, n, r_inertial, q_inertial2body)

% Down in body frame
down_inertial = -r_inertial/norm(r_inertial);
down_body = QuatTransform(q_inertial2body,down_inertial);

% Gravity gradient torque
T = 3*n^2*cross(down_body,J*down_body);

== matlab function project_sim/Plant/Attitude Dynamics/MATLAB Function ==
  data: omega input; q_dot output; q input
function q_dot = QuaternionEvolution(omega, q)
intermed = [omega; 0];
q_dot = 0.5*QuatProduct(intermed,q);

== matlab function project_sim/Plant/Gravity Gradient Torque/MATLAB Function ==
  data: mu input; n output; r input
function n = OrbitRate(mu,r)

n = sqrt(mu/norm(r)^3);

== matlab function project_sim/Flight Software/Gravity Gradient Torque/GG Torque Computation ==
  data: J input; T output; n input; r_inertial input; q_inertial2body input
function T = GGTorque(J, n, r_inertial, q_inertial2body)

% Down in body frame
down_inertial = -r_inertial/norm(r_inertial);
down_body = QuatTransform(q_inertial2body,down_inertial);

% Gravity gradient torque
T = 3*n^2*cross(down_body,J*down_body);

== matlab function project_sim/Flight Software/Gravity Gradient Torque/MATLAB Function ==
  data: mu input; n output; r input
function n = OrbitRate(mu,r)

n = sqrt(mu/norm(r)^3);

== matlab function project_sim/Actuator/MATLAB Function ==
  data: h0 input; h output; theta input
function h = CMG_AngMom(h0, theta)
% Produces the angular momentum vector for the CMGs

% Extract alpha and betas
alphas = theta(1:4);
betas = theta(5:8);

h = zeros(3,1);
for ii = 1:4
    h = h + h0*[sin(alphas(ii)); cos(alphas(ii))*cos(betas(ii)); cos(alphas(ii))*sin(betas(ii))];
end

== matlab function project_sim/Actuator/MATLAB Function1 ==
  data: X output; theta input
function X = CMG_X(theta)
% Produces the matrix of CMG spin axes

% Extract alpha and betas
alphas = theta(1:4);
betas = theta(5:8);

X = zeros(3,8);
for ii = 1:4
    X(:,2*ii-1:2*ii) = [cos(alphas(ii)), 0;
        -sin(alphas(ii))*cos(betas(ii)), -cos(alphas(ii))*sin(betas(ii));
        -sin(alphas(ii))*sin(betas(ii)), cos(alphas(ii))*cos(betas(ii))];
end

== matlab function project_sim/Flight Software/Nonlinear PD Controller/MATLAB Function ==
  data: u input; y output; v input
function y = CrossProduct(u,v)

y = CrossProductMat(u)*v;

== matlab function project_sim/Actuator/MATLAB Function2 ==
  data: u input; y output; v input
function y = CrossProduct(u,v)

y = CrossProductMat(u)*v;

== matlab function project_sim/MATLAB Function ==
  data: q input; q_pet output; a input
function q_pet = PeturbQuaternion(q, a)

% Convert a to dq
dq = [0.5*a; 1];
dq = dq/norm(dq);

% Peturb
q_pet = QuatProduct(dq,q);

== matlab function project_sim/Flight Software/Attitude Estimation/Propagation ==
  data: q_inertial2body input; q_inertial2body_new output; w_body input; Phat input; J input; dt input; w_body_new output; Phat_new output; Q input; u input
function [q_inertial2body_new, w_body_new, Phat_new] = fcn(q_inertial2body, w_body, Phat, J, dt, Q, u)

% Propagate Attitude
[q_inertial2body_new, w_body_new] = AttitudePropagate(q_inertial2body, w_body, J, dt, "RK4",u);

% Propagate Covariance
Aeval = PaPaFunc(dt,...
    w_body(1),...
    w_body(2),...
    w_body(3)+1E-10); % Add very small peturbation to prevent divide by zero
Beval = PaPdomegaFunc(dt,...
    w_body(1),...
    w_body(2),...
    w_body(3)+1E-10); % Add very small peturbation to prevent divide by zero
F = [ Aeval, Beval;
    zeros(3), eye(3)];
Phat_new = F*Phat*F' + Q;

end

== matlab function project_sim/Plant/Position Dynamics/Vector Norm ==
  data: r input; a output; mu input
function a = TwoBodyGrav(r,mu)

nr = norm(r);
a = -mu*r/(nr^3);

== matlab function project_sim/Flight Software/Attitude Estimation/MEKF Update ==
  data: q_inertial2body_est output; q_inertial2body_meas input; w_body_meas input; q_inertial2body_pred input; w_pred input; Phat_pred input; w_est output; Phat output; R_a input; R_w input; underweight input
function [q_inertial2body_est, w_est, Phat] = Update(q_inertial2body_meas, w_body_meas, q_inertial2body_pred, w_pred, Phat_pred, R_a, R_w, underweight)

% Find the error quaternion
dq = QuatProduct(q_inertial2body_meas,QuatInv(q_inertial2body_pred));
a_meas = 2*dq(1:3);

% Jacobian for direct measurement of a and w
H = [eye(3), zeros(3);
    zeros(3), eye(3)];

% Kalman gain
R = blkdiag(R_a,R_w);
K = Phat_pred*H'/((1+underweight)*H*Phat_pred*H' + R);

% update
xbar = [zeros(3,1); w_pred];
xhat = xbar + K*([a_meas; w_body_meas] - H*xbar);
w_est = xhat(4:6);

% Apply update to quaternion
dqhat = [xhat(1:3); 1];
dqhat = dqhat/norm(dqhat);
q_inertial2body_est = QuatProduct(dqhat,q_inertial2body_pred);

% Update covariance
Phat = (eye(6) - K*H)*Phat_pred*(eye(6) - K*H)' + K*R*K';

end

== matlab function project_sim/Plant/Attitude Dynamics/MATLAB Function1 ==
  data: J input; omega_dot output; T input; omega input
function omega_dot = OmegaEvolution(J, T, omega)
omega_dot = J\(T - cross(omega, J*omega));

== matlab function project_sim/Plant/Attitude Dynamics/Vector Normalize ==
  data: v input; nv output
function nv = NormVec(v)

nv = v/norm(v);

== matlab function project_sim/Flight Software/Inertial Reference/Inertial To LVLH Dynamics/Attitude Dynamics/MATLAB Function ==
  data: omega input; q_dot output; q input
function q_dot = QuaternionEvolution(omega, q)
intermed = [omega; 0];
q_dot = 0.5*QuatProduct(intermed,q);

== matlab function project_sim/Flight Software/Inertial Reference/Inertial To LVLH Dynamics/Attitude Dynamics/MATLAB Function1 ==
  data: J input; omega_dot output; T input; omega input
function omega_dot = OmegaEvolution(J, T, omega)
omega_dot = J\(T - cross(omega, J*omega));

== matlab function project_sim/Flight Software/Inertial Reference/Inertial To LVLH Dynamics/Attitude Dynamics/Vector Normalize ==
  data: v input; nv output
function nv = NormVec(v)

nv = v/norm(v);

== matlab function project_sim/Flight Software/Estimated Pointing and Rate Errors/MATLAB Function ==
  data: q_inertial2body_ref input; q_ref2actual output; q_inertial2body_actual input
function q_ref2actual = ErrorQuat(q_inertial2body_ref, q_inertial2body_actual)

q_ref2actual = QuatProduct(q_inertial2body_actual,QuatInv(q_inertial2body_ref));

% Force normalization
q_ref2actual = q_ref2actual/norm(q_ref2actual);

== matlab function project_sim/Flight Software/Estimated Pointing and Rate Errors/MATLAB Function1 ==
  data: w_ref input; delta_w output; w_actual input; q_ref2actual input
function delta_w = ErrorRate(w_ref, w_actual, q_ref2actual)

delta_w = w_actual - QuatTransform(q_ref2actual,w_ref);

== matlab function project_sim/Flight Software/Estimated Pointing and Rate Errors/MATLAB Function2 ==
  data: q_err input; dtheta output
function dtheta = ErrorQuat2ErrorAngle(q_err)

% Quaternion components
q_v = real(q_err(1:3));
q_s = real(q_err(4));

dtheta = [atan2(q_v(1),q_s);
    atan2(q_v(2),q_s);
    atan2(q_v(3),q_s)];

== matlab function project_sim/Flight Software/Estimated Pointing and Rate Errors/MATLAB Function3 ==
  data: omega_ref input; dthetadot output; delta_omega input; delta_theta input
function dthetadot = ErrorThetaDot(omega_ref, delta_omega, delta_theta)

dthetadot = delta_omega - cross(omega_ref,delta_theta);
